simulink model "zuoti3_6_"  (R2022a)
settings: Solver=VariableStepAuto  StartTime=0.0  StopTime=10.0  RelTol=1e-3
libraries: spsSeriesRLCBranchLib x16, spsControlledCurrentSourceLib x1, spsCurrentMeasurementLib x1, spspowerguiLib x1
settings Model: Creator=Rov  LastModifiedBy=Rov

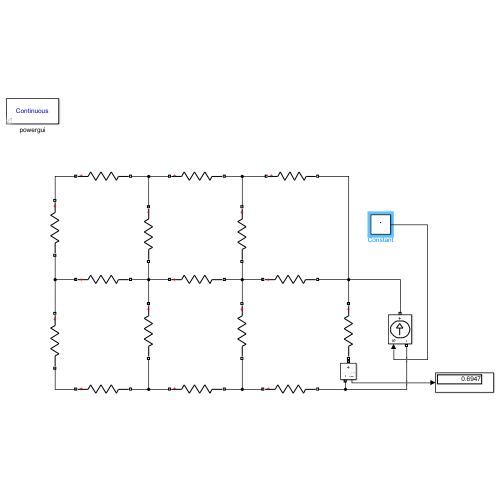
[thumbnail: Simulink's stored preview of the top-level diagram]
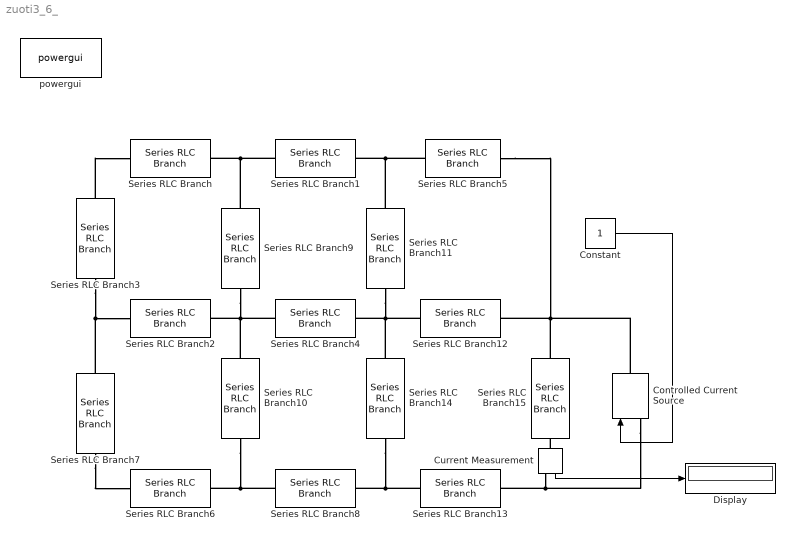
== system zuoti3_6_ ==
  Constant : Constant
  Controlled Current Source : spsControlledCurrentSourceLib/Controlled Current Source  Initialize=off  Source_Type=DC  Amplitude=0  Phase=0  Frequency=0  Measurements=None
  Current Measurement : spsCurrentMeasurementLib/Current Measurement  PhasorSimulation=off  OutputType=Complex  PSBequivalent=0
  Display : Display
  Series RLC Branch{,1..15} (16 alike) : spsSeriesRLCBranchLib/Series RLC Branch  LConnTagsString=__new0  RConnTagsString=__new0  BranchType=R  Resistance=1  Inductance=1e-3  SetiL0=off  InitialCurrent=0  Capacitance=1e-6  Setx0=off  InitialVoltage=0  Measurements=None
  powergui : spspowerguiLib/powergui  Priority=1  SimulationMode=Continuous  SampleTime=50e-6  frequency=60  Iterations=50  frequencyindice=0  Pbase=100e6  ErrMax=1e-4  UnitsV=kV  UnitsW=MW  buscounter=0  FunctionMessages=off  echomessages=off  EnableUseOfTLC=off  CurrentSourceSwitches=off  DisableSnubberDevices=off  DisableRonSwitches=off  DisableVfSwitches=off  DisplayEquations=off  AutomaticDiscreteSolvers=off  SolverType=Tustin/Backward Euler (TBE)  Interpol=off  ExternalGateDelay=off  methode=off  Ts=100  x0status=blocks  SPID=on  SwTol=0  HookPort=off  NonlinearTolerance=1e-4  nMaxIteration=100  ContinueOnMaxIteration=off  RestoreLinks=warning  ResistiveCurrentMeasurement=off  Frange=[0:2:500]  Ylog=off  Xlog=on  ShowGrid=off  save=off  variable=ZData  structure=0  ZoomFFT=off  StartTime=0.0  cycles=1  DisplayStyle=1  fundamental=60  FreqAxis=off  MaxFrequency=1000  frequencyindicesteady=1  RmsSteady=1  display=off
  wires:
  Constant/1 -> Controlled Current Source/1
  Current Measurement/1 -> Display/1
  connections:
  Series RLC Branch1/LConn1 -- Series RLC Branch9/LConn1 -- Series RLC Branch/RConn1
  Series RLC Branch3/LConn1 -- Series RLC Branch/LConn1
  Series RLC Branch3/RConn1 -- Series RLC Branch7/LConn1 -- Series RLC Branch2/LConn1
  Series RLC Branch4/LConn1 -- Series RLC Branch10/LConn1 -- Series RLC Branch9/RConn1 -- Series RLC Branch2/RConn1
  Series RLC Branch5/LConn1 -- Series RLC Branch11/LConn1 -- Series RLC Branch1/RConn1
  Series RLC Branch8/LConn1 -- Series RLC Branch10/RConn1 -- Series RLC Branch6/RConn1
  Series RLC Branch7/RConn1 -- Series RLC Branch6/LConn1
  Series RLC Branch12/LConn1 -- Series RLC Branch4/RConn1 -- Series RLC Branch14/LConn1 -- Series RLC Branch11/RConn1
  Series RLC Branch13/LConn1 -- Series RLC Branch14/RConn1 -- Series RLC Branch8/RConn1
  Series RLC Branch15/LConn1 -- Controlled Current Source/RConn1 -- Series RLC Branch5/RConn1 -- Series RLC Branch12/RConn1
  Controlled Current Source/LConn1 -- Series RLC Branch13/RConn1 -- Current Measurement/RConn1
  Current Measurement/LConn1 -- Series RLC Branch15/RConn1
